simulink model "Drone_Formation"  (R2025a)
settings: Solver=FixedStepAuto  StartTime=0.0  StopTime=50  FixedStep=0.01  RelTol=1e-3
(part 1 of 2)
settings Model: Creator=huy01  LastModifiedBy=huy01

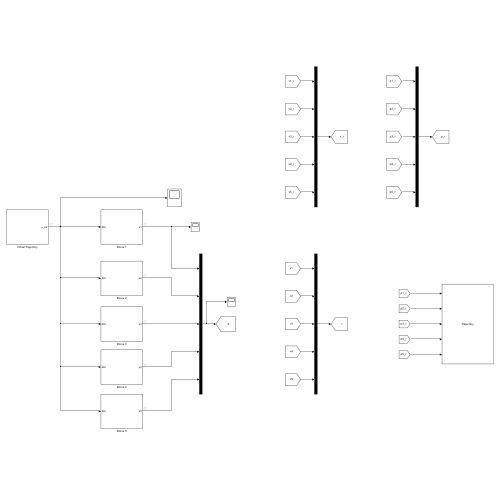
[thumbnail: Simulink's stored preview of the top-level diagram]
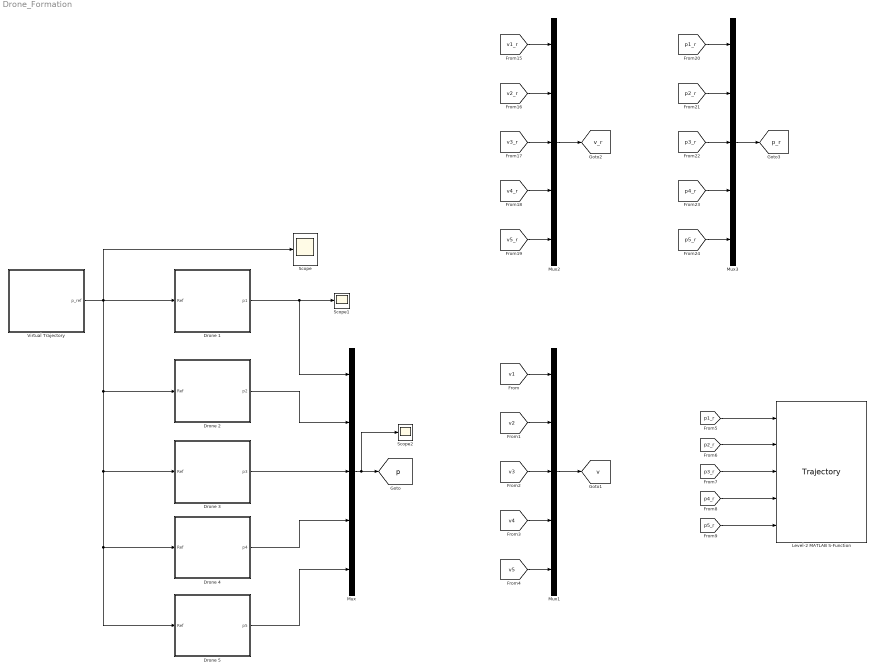
== system Drone_Formation ==
  Drone 1 : Subsystem
  Drone 2 : Subsystem
  Drone 3 : Subsystem
  Drone 4 : Subsystem
  Drone 5 : Subsystem
  Level-2 MATLAB S-Function : M-S-Function  FunctionName=Trajectory
  Mux{,1..3} (4 alike) : Mux  Inputs=5
  Scope : Scope
      settings: ActiveDisplayYMaximum=40
  Scope1 : Scope
      settings: ActiveDisplayYMinimum=-1380.4300146371204  ActiveDisplayYMaximum=836.3107963286418
  Scope2 : Scope
      settings: ActiveDisplayYMinimum=-1  ActiveDisplayYMaximum=1  DataLoggingVariableName=ScopeData2
  Virtual Trajectory : Subsystem
  tag scope: p=global, p_r=global, v=global, v_r=global
  wires:
  Virtual Trajectory/1(p_ref) -> Scope/1, Drone 1/1(Ref), Drone 2/1(Ref), Drone 5/1(Ref), Drone 4/1(Ref), Drone 3/1(Ref)
  Drone 3/1(p3) -> Mux/3
  Drone 4/1(p4) -> Mux/4
  Drone 5/1(p5) -> Mux/5
  Drone 1/1(p1) -> Scope1/1, Mux/1
  Drone 2/1(p2) -> Mux/2
  Mux/1 -> Scope2/1, [p]
  [v1] -> Mux1/1
  [v2] -> Mux1/2
  [v3] -> Mux1/3
  [v4] -> Mux1/4
  [v5] -> Mux1/5
  Mux1/1 -> [v]
  [p2_r] -> Level-2 MATLAB S-Function/2
  [p3_r] -> Level-2 MATLAB S-Function/3
  [p4_r] -> Level-2 MATLAB S-Function/4
  [p5_r] -> Level-2 MATLAB S-Function/5
  [p1_r] -> Level-2 MATLAB S-Function/1
  Mux2/1 -> [v_r]
  [v5_r] -> Mux2/5
  [v1_r] -> Mux2/1
  [v2_r] -> Mux2/2
  [v4_r] -> Mux2/4
  [v3_r] -> Mux2/3
  Mux3/1 -> [p_r]
  [p5_r] -> Mux3/5
  [p1_r] -> Mux3/1
  [p2_r] -> Mux3/2
  [p4_r] -> Mux3/4
  [p3_r] -> Mux3/3

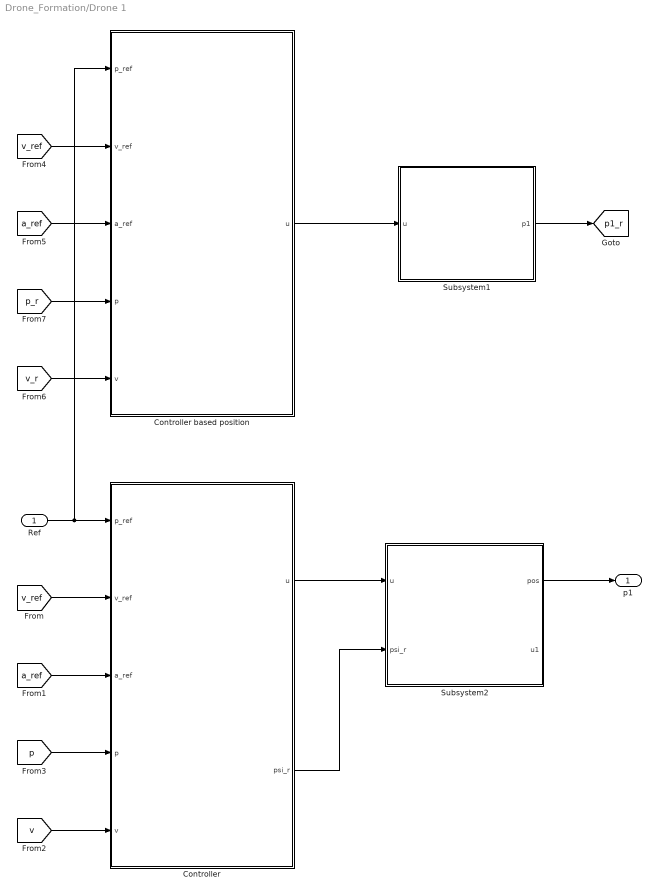
== system Drone_Formation/Drone 1 ==
  Ref : Inport
  Controller : MATLAB Function  TreatAsAtomicUnit=on
  Controller based position : MATLAB Function  TreatAsAtomicUnit=on
  Subsystem1 : Subsystem
  Subsystem2 : Subsystem
  p1 : Outport
  tag scope: p1_r=global
  wires:
  Ref/1 -> Controller based position/1(p_ref), Controller/1(p_ref)
  [v_ref] -> Controller/2(v_ref)
  [a_ref] -> Controller/3(a_ref)
  [v] -> Controller/5(v)
  [p] -> Controller/4(p)
  Controller/1(u) -> Subsystem2/1(u)
  Controller/2(psi_r) -> Subsystem2/2(psi_r)
  Subsystem2/1(pos) -> p1/1
  Subsystem1/1(p1) -> [p1_r]
  [a_ref] -> Controller based position/3(a_ref)
  [v_r] -> Controller based position/5(v)
  [p_r] -> Controller based position/4(p)
  Controller based position/1(u) -> Subsystem1/1(u)
  [v_ref] -> Controller based position/2(v_ref)

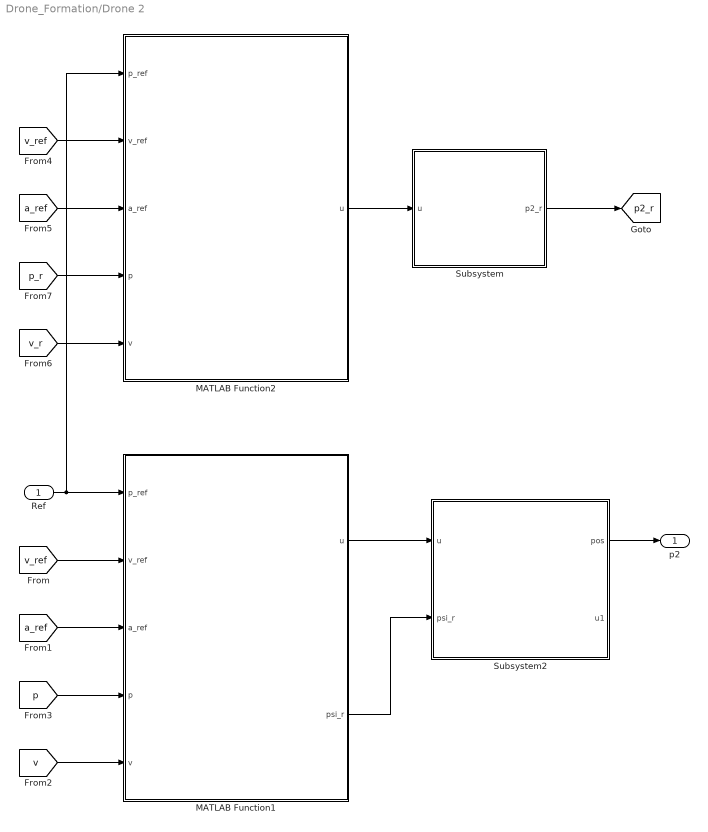
== system Drone_Formation/Drone 2 ==
  Ref : Inport
  MATLAB Function1 : MATLAB Function  TreatAsAtomicUnit=on
  MATLAB Function2 : MATLAB Function  TreatAsAtomicUnit=on
  Subsystem : Subsystem
  Subsystem2 : Subsystem
  p2 : Outport
  tag scope: p2_r=global
  wires:
  [v_ref] -> MATLAB Function1/2(v_ref)
  [a_ref] -> MATLAB Function1/3(a_ref)
  [v] -> MATLAB Function1/5(v)
  [p] -> MATLAB Function1/4(p)
  MATLAB Function1/1(u) -> Subsystem2/1(u)
  MATLAB Function1/2(psi_r) -> Subsystem2/2(psi_r)
  Subsystem2/1(pos) -> p2/1
  Subsystem/1(p2_r) -> [p2_r]
  MATLAB Function2/1(u) -> Subsystem/1(u)
  Ref/1 -> MATLAB Function2/1(p_ref), MATLAB Function1/1(p_ref)
  [v_ref] -> MATLAB Function2/2(v_ref)
  [v_r] -> MATLAB Function2/5(v)
  [p_r] -> MATLAB Function2/4(p)
  [a_ref] -> MATLAB Function2/3(a_ref)

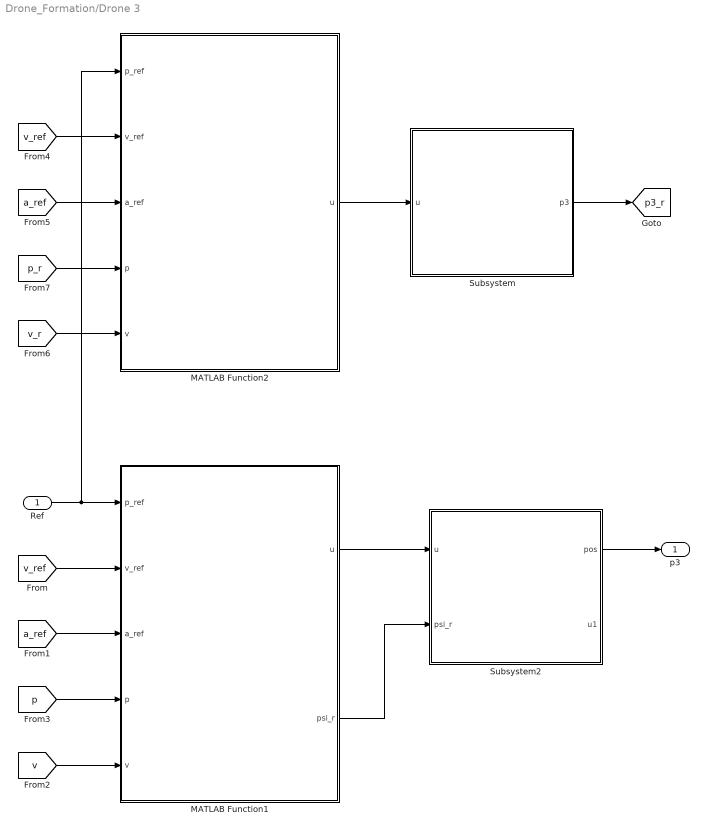
== system Drone_Formation/Drone 3 ==
  Ref : Inport
  MATLAB Function1 : MATLAB Function  TreatAsAtomicUnit=on
  MATLAB Function2 : MATLAB Function  TreatAsAtomicUnit=on
  Subsystem : Subsystem
  Subsystem2 : Subsystem
  p3 : Outport
  tag scope: p3_r=global
  wires:
  Ref/1 -> MATLAB Function2/1(p_ref), MATLAB Function1/1(p_ref)
  [v_ref] -> MATLAB Function1/2(v_ref)
  [a_ref] -> MATLAB Function1/3(a_ref)
  [v] -> MATLAB Function1/5(v)
  [p] -> MATLAB Function1/4(p)
  MATLAB Function1/1(u) -> Subsystem2/1(u)
  MATLAB Function1/2(psi_r) -> Subsystem2/2(psi_r)
  Subsystem2/1(pos) -> p3/1
  Subsystem/1(p3) -> [p3_r]
  [v_ref] -> MATLAB Function2/2(v_ref)
  [a_ref] -> MATLAB Function2/3(a_ref)
  [v_r] -> MATLAB Function2/5(v)
  [p_r] -> MATLAB Function2/4(p)
  MATLAB Function2/1(u) -> Subsystem/1(u)

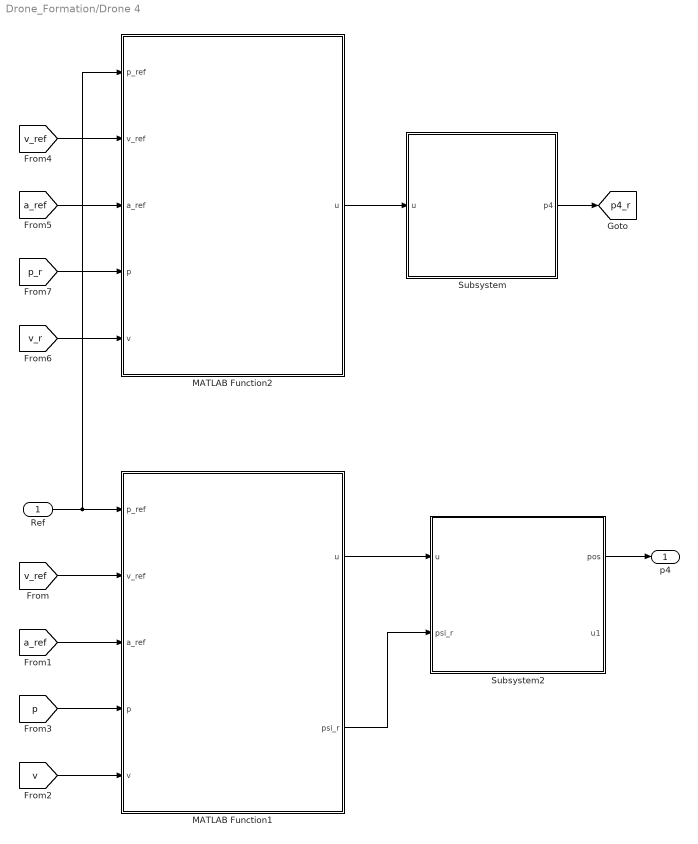
== system Drone_Formation/Drone 4 ==
  Ref : Inport
  MATLAB Function1 : MATLAB Function  TreatAsAtomicUnit=on
  MATLAB Function2 : MATLAB Function  TreatAsAtomicUnit=on
  Subsystem : Subsystem
  Subsystem2 : Subsystem
  p4 : Outport
  tag scope: p4_r=global
  wires:
  Ref/1 -> MATLAB Function2/1(p_ref), MATLAB Function1/1(p_ref)
  [v_ref] -> MATLAB Function1/2(v_ref)
  [a_ref] -> MATLAB Function1/3(a_ref)
  [v] -> MATLAB Function1/5(v)
  [p] -> MATLAB Function1/4(p)
  MATLAB Function1/1(u) -> Subsystem2/1(u)
  MATLAB Function1/2(psi_r) -> Subsystem2/2(psi_r)
  Subsystem2/1(pos) -> p4/1
  Subsystem/1(p4) -> [p4_r]
  [a_ref] -> MATLAB Function2/3(a_ref)
  [p_r] -> MATLAB Function2/4(p)
  [v_ref] -> MATLAB Function2/2(v_ref)
  [v_r] -> MATLAB Function2/5(v)
  MATLAB Function2/1(u) -> Subsystem/1(u)

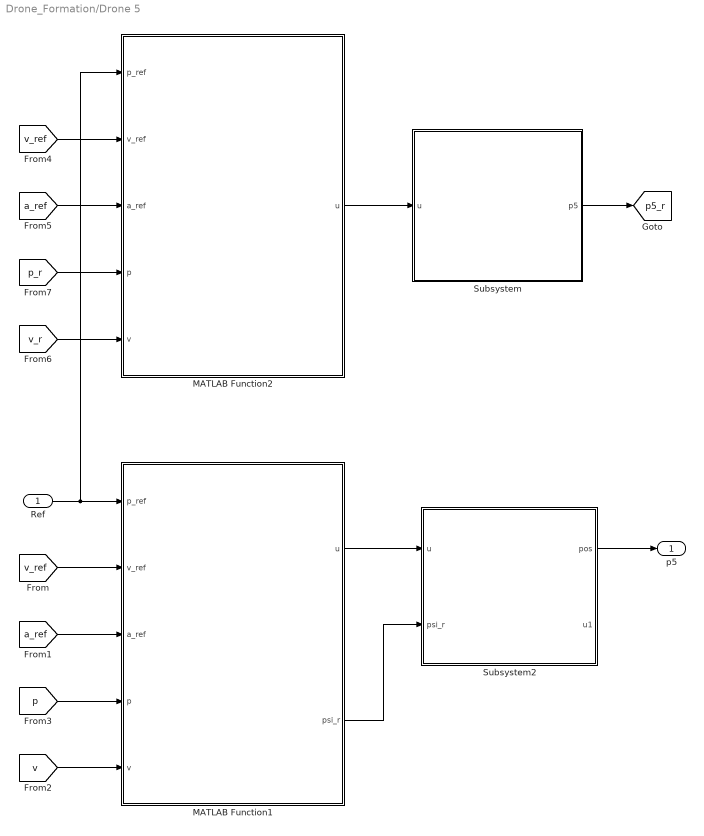
== system Drone_Formation/Drone 5 ==
  Ref : Inport
  MATLAB Function1 : MATLAB Function  TreatAsAtomicUnit=on
  MATLAB Function2 : MATLAB Function  TreatAsAtomicUnit=on
  Subsystem : Subsystem
  Subsystem2 : Subsystem
  p5 : Outport
  tag scope: p5_r=global
  wires:
  Ref/1 -> MATLAB Function2/1(p_ref), MATLAB Function1/1(p_ref)
  [v_ref] -> MATLAB Function1/2(v_ref)
  [a_ref] -> MATLAB Function1/3(a_ref)
  [v] -> MATLAB Function1/5(v)
  [p] -> MATLAB Function1/4(p)
  MATLAB Function1/1(u) -> Subsystem2/1(u)
  MATLAB Function1/2(psi_r) -> Subsystem2/2(psi_r)
  Subsystem2/1(pos) -> p5/1
  Subsystem/1(p5) -> [p5_r]
  [a_ref] -> MATLAB Function2/3(a_ref)
  [v_ref] -> MATLAB Function2/2(v_ref)
  [p_r] -> MATLAB Function2/4(p)
  [v_r] -> MATLAB Function2/5(v)
  MATLAB Function2/1(u) -> Subsystem/1(u)

== system Drone_Formation/Virtual Trajectory ==
  Clock : Clock
  Derivative : Derivative
  Derivative1 : Derivative
  MATLAB Function : MATLAB Function  TreatAsAtomicUnit=on
  p_ref : Outport
  tag scope: a_ref=global, v_ref=global
  wires:
  MATLAB Function/1(p_ref) -> Derivative/1, p_ref/1
  Clock/1 -> MATLAB Function/1(t)
  Derivative/1 -> Derivative1/1, [v_ref]
  Derivative1/1 -> [a_ref]

== system Drone_Formation/Drone 1/Subsystem1 ==
  u : Inport
  Integrator : Integrator  InitialCondition=zeros(3,1)
  Integrator1 : Integrator  InitialCondition=[4;5;0];
  Kinematic : MATLAB Function  TreatAsAtomicUnit=on
  p1 : Outport
  tag scope: v1_r=global
  wires:
  Integrator1/1 -> p1/1
  u/1 -> Kinematic/1(u)
  Integrator/1 -> [v1_r], Integrator1/1
  Kinematic/1(p1_ddot) -> Integrator/1

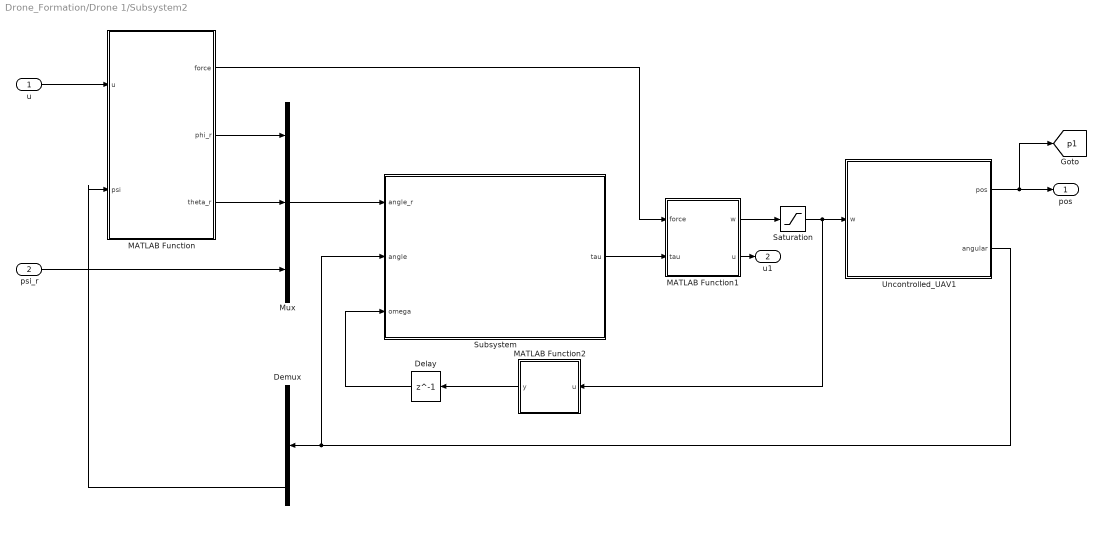
== system Drone_Formation/Drone 1/Subsystem2 ==
  u : Inport
  psi_r : Inport  Port=2
  Delay : Delay  DelayLength=1  InputProcessing=Columns as channels (frame based)
  Demux : Demux  Outputs=3
  MATLAB Function : MATLAB Function  TreatAsAtomicUnit=on
  MATLAB Function1 : MATLAB Function  TreatAsAtomicUnit=on
  MATLAB Function2 : MATLAB Function  TreatAsAtomicUnit=on
  Mux : Mux  Inputs=3
  Saturation : Saturate  UpperLimit=2300  LowerLimit=0
  Subsystem : Subsystem
  Uncontrolled_UAV1 : Subsystem
  pos : Outport
  u1 : Outport  Port=2
  tag scope: p1=global
  wires:
  MATLAB Function/2(phi_r) -> Mux/1
  Mux/1 -> Subsystem/1(angle_r)
  Uncontrolled_UAV1/2(angular) -> Subsystem/2(angle), Demux/1
  Saturation/1 -> Uncontrolled_UAV1/1(w), MATLAB Function2/1(u)
  MATLAB Function/3(theta_r) -> Mux/2
  Delay/1 -> Subsystem/3(omega)
  Subsystem/1(tau) -> MATLAB Function1/2(tau)
  psi_r/1 -> Mux/3
  MATLAB Function2/1(y) -> Delay/1
  MATLAB Function1/1(w) -> Saturation/1
  Demux/3 -> MATLAB Function/2(psi)
  MATLAB Function/1(force) -> MATLAB Function1/1(force)
  Uncontrolled_UAV1/1(pos) -> [p1], pos/1
  u/1 -> MATLAB Function/1(u)
  MATLAB Function1/2(u) -> u1/1

== system Drone_Formation/Drone 2/Subsystem ==
  u : Inport
  Integrator : Integrator  InitialCondition=zeros(3,1)
  Integrator1 : Integrator  InitialCondition=[5;1;0];
  Kinematic : MATLAB Function  TreatAsAtomicUnit=on
  p2_r : Outport
  tag scope: v2_r=global
  wires:
  Integrator/1 -> [v2_r], Integrator1/1
  Integrator1/1 -> p2_r/1
  u/1 -> Kinematic/1(u)
  Kinematic/1(p1_ddot) -> Integrator/1

== system Drone_Formation/Drone 2/Subsystem2 ==
  u : Inport
  psi_r : Inport  Port=2
  Delay : Delay  DelayLength=1  InputProcessing=Columns as channels (frame based)
  Demux : Demux  Outputs=3
  MATLAB Function : MATLAB Function  TreatAsAtomicUnit=on
  MATLAB Function1 : MATLAB Function  TreatAsAtomicUnit=on
  MATLAB Function2 : MATLAB Function  TreatAsAtomicUnit=on
  Mux : Mux  Inputs=3
  Saturation : Saturate  UpperLimit=2300  LowerLimit=0
  Subsystem : Subsystem
  Uncontrolled_UAV1 : Subsystem
  pos : Outport
  u1 : Outport  Port=2
  tag scope: p2=global
  wires:
  MATLAB Function/2(phi_r) -> Mux/1
  Mux/1 -> Subsystem/1(angle_r)
  Uncontrolled_UAV1/2(angular) -> Subsystem/2(angle), Demux/1
  Saturation/1 -> Uncontrolled_UAV1/1(w), MATLAB Function2/1(u)
  MATLAB Function/3(theta_r) -> Mux/2
  Delay/1 -> Subsystem/3(omega)
  Subsystem/1(tau) -> MATLAB Function1/2(tau)
  psi_r/1 -> Mux/3
  MATLAB Function2/1(y) -> Delay/1
  MATLAB Function1/1(w) -> Saturation/1
  Demux/3 -> MATLAB Function/2(psi)
  MATLAB Function/1(force) -> MATLAB Function1/1(force)
  Uncontrolled_UAV1/1(pos) -> [p2], pos/1
  u/1 -> MATLAB Function/1(u)
  MATLAB Function1/2(u) -> u1/1

== system Drone_Formation/Drone 3/Subsystem ==
  u : Inport
  Integrator : Integrator  InitialCondition=zeros(3,1)
  Integrator1 : Integrator  InitialCondition=zeros(3,1)
  Kinematic : MATLAB Function  TreatAsAtomicUnit=on
  p3 : Outport
  tag scope: v3_r=global
  wires:
  u/1 -> Kinematic/1(u)
  Integrator1/1 -> p3/1
  Integrator/1 -> [v3_r], Integrator1/1
  Kinematic/1(p1_ddot) -> Integrator/1

== system Drone_Formation/Drone 3/Subsystem2 ==
  u : Inport
  psi_r : Inport  Port=2
  Delay : Delay  DelayLength=1  InputProcessing=Columns as channels (frame based)
  Demux : Demux  Outputs=3
  MATLAB Function : MATLAB Function  TreatAsAtomicUnit=on
  MATLAB Function1 : MATLAB Function  TreatAsAtomicUnit=on
  MATLAB Function2 : MATLAB Function  TreatAsAtomicUnit=on
  Mux : Mux  Inputs=3
  Saturation : Saturate  UpperLimit=2300  LowerLimit=0
  Subsystem : Subsystem
  Uncontrolled_UAV1 : Subsystem
  pos : Outport
  u1 : Outport  Port=2
  tag scope: p3=global
  wires:
  MATLAB Function/2(phi_r) -> Mux/1
  Mux/1 -> Subsystem/1(angle_r)
  Uncontrolled_UAV1/2(angular) -> Subsystem/2(angle), Demux/1
  Saturation/1 -> Uncontrolled_UAV1/1(w), MATLAB Function2/1(u)
  MATLAB Function/3(theta_r) -> Mux/2
  Delay/1 -> Subsystem/3(omega)
  Subsystem/1(tau) -> MATLAB Function1/2(tau)
  psi_r/1 -> Mux/3
  MATLAB Function2/1(y) -> Delay/1
  MATLAB Function1/1(w) -> Saturation/1
  Demux/3 -> MATLAB Function/2(psi)
  MATLAB Function/1(force) -> MATLAB Function1/1(force)
  Uncontrolled_UAV1/1(pos) -> [p3], pos/1
  u/1 -> MATLAB Function/1(u)
  MATLAB Function1/2(u) -> u1/1

== system Drone_Formation/Drone 4/Subsystem ==
  u : Inport
  Integrator : Integrator  InitialCondition=zeros(3,1)
  Integrator1 : Integrator  InitialCondition=[10;2;0];
  Kinematic : MATLAB Function  TreatAsAtomicUnit=on
  p4 : Outport
  tag scope: v4_r=global
  wires:
  Integrator1/1 -> p4/1
  Integrator/1 -> [v4_r], Integrator1/1
  Kinematic/1(p1_ddot) -> Integrator/1
  u/1 -> Kinematic/1(u)

== system Drone_Formation/Drone 4/Subsystem2 ==
  u : Inport
  psi_r : Inport  Port=2
  Delay : Delay  DelayLength=1  InputProcessing=Columns as channels (frame based)
  Demux : Demux  Outputs=3
  MATLAB Function : MATLAB Function  TreatAsAtomicUnit=on
  MATLAB Function1 : MATLAB Function  TreatAsAtomicUnit=on
  MATLAB Function2 : MATLAB Function  TreatAsAtomicUnit=on
  Mux : Mux  Inputs=3
  Saturation : Saturate  UpperLimit=2300  LowerLimit=0
  Subsystem : Subsystem
  Uncontrolled_UAV1 : Subsystem
  pos : Outport
  u1 : Outport  Port=2
  tag scope: p4=global
  wires:
  MATLAB Function/2(phi_r) -> Mux/1
  Mux/1 -> Subsystem/1(angle_r)
  Uncontrolled_UAV1/2(angular) -> Subsystem/2(angle), Demux/1
  Saturation/1 -> Uncontrolled_UAV1/1(w), MATLAB Function2/1(u)
  MATLAB Function/3(theta_r) -> Mux/2
  Delay/1 -> Subsystem/3(omega)
  Subsystem/1(tau) -> MATLAB Function1/2(tau)
  psi_r/1 -> Mux/3
  MATLAB Function2/1(y) -> Delay/1
  MATLAB Function1/1(w) -> Saturation/1
  Demux/3 -> MATLAB Function/2(psi)
  MATLAB Function/1(force) -> MATLAB Function1/1(force)
  Uncontrolled_UAV1/1(pos) -> [p4], pos/1
  u/1 -> MATLAB Function/1(u)
  MATLAB Function1/2(u) -> u1/1

== system Drone_Formation/Drone 5/Subsystem ==
  u : Inport
  Integrator : Integrator  InitialCondition=zeros(3,1)
  Integrator1 : Integrator  InitialCondition=[15;0;0];
  Kinematic : MATLAB Function  TreatAsAtomicUnit=on
  p5 : Outport
  tag scope: v5_r=global
  wires:
  Integrator1/1 -> p5/1
  Kinematic/1(p1_ddot) -> Integrator/1
  Integrator/1 -> [v5_r], Integrator1/1
  u/1 -> Kinematic/1(u)

== system Drone_Formation/Drone 5/Subsystem2 ==
  u : Inport
  psi_r : Inport  Port=2
  Delay : Delay  DelayLength=1  InputProcessing=Columns as channels (frame based)
  Demux : Demux  Outputs=3
  MATLAB Function : MATLAB Function  TreatAsAtomicUnit=on
  MATLAB Function1 : MATLAB Function  TreatAsAtomicUnit=on
  MATLAB Function2 : MATLAB Function  TreatAsAtomicUnit=on
  Mux : Mux  Inputs=3
  Saturation : Saturate  UpperLimit=2300  LowerLimit=0
  Subsystem : Subsystem
  Uncontrolled_UAV1 : Subsystem
  pos : Outport
  u1 : Outport  Port=2
  tag scope: p5=global
  wires:
  MATLAB Function/2(phi_r) -> Mux/1
  Mux/1 -> Subsystem/1(angle_r)
  Uncontrolled_UAV1/2(angular) -> Subsystem/2(angle), Demux/1
  Saturation/1 -> Uncontrolled_UAV1/1(w), MATLAB Function2/1(u)
  MATLAB Function/3(theta_r) -> Mux/2
  Delay/1 -> Subsystem/3(omega)
  Subsystem/1(tau) -> MATLAB Function1/2(tau)
  psi_r/1 -> Mux/3
  MATLAB Function2/1(y) -> Delay/1
  MATLAB Function1/1(w) -> Saturation/1
  Demux/3 -> MATLAB Function/2(psi)
  MATLAB Function/1(force) -> MATLAB Function1/1(force)
  Uncontrolled_UAV1/1(pos) -> [p5], pos/1
  u/1 -> MATLAB Function/1(u)
  MATLAB Function1/2(u) -> u1/1

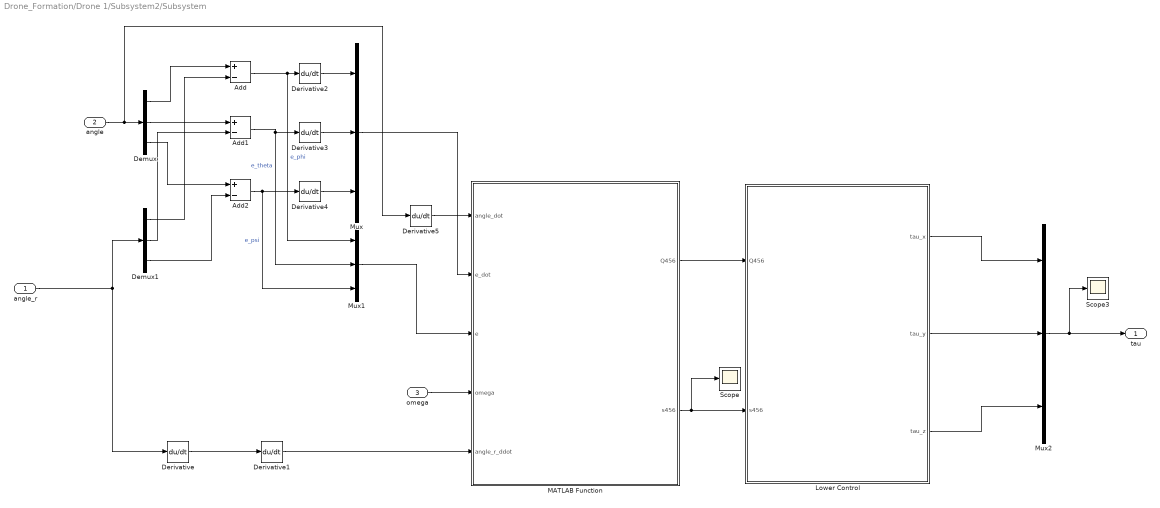
== system Drone_Formation/Drone 1/Subsystem2/Subsystem ==
  angle_r : Inport
  angle : Inport  Port=2
  omega : Inport  Port=3
  Add : Sum  Inputs=+-
  Add1 : Sum  Inputs=+-
  Add2 : Sum  Inputs=+-
  Demux : Demux  Outputs=3
  Demux1 : Demux  Outputs=3
  Derivative{,1..5} (6 alike) : Derivative
  Lower Control : MATLAB Function  TreatAsAtomicUnit=on
  MATLAB Function : MATLAB Function  TreatAsAtomicUnit=on
  Mux : Mux  Inputs=3
  Mux1 : Mux  Inputs=3
  Mux2 : Mux  Inputs=3
  Scope : Scope
      settings: ActiveDisplayYMinimum=-354.73382878164716  ActiveDisplayYMaximum=368.3791602340649  DataLoggingVariableName=ScopeData22
  Scope3 : Scope
      settings: ActiveDisplayYMinimum=-334.14921407033052  ActiveDisplayYMaximum=201.68653412472139  DataLoggingVariableName=ScopeData11
  tau : Outport
  wires:
  Add2/1 -> Mux1/3, Derivative4/1  "e_psi"
  Lower Control/2(tau_y) -> Mux2/2
  Mux1/1 -> MATLAB Function/3(e)
  Mux/1 -> MATLAB Function/2(e_dot)
  Mux2/1 -> tau/1, Scope3/1
  omega/1 -> MATLAB Function/4(omega)
  Add/1 -> Mux1/1, Derivative2/1  "e_phi"
  angle/1 -> Derivative5/1, Demux/1
  Derivative1/1 -> MATLAB Function/5(angle_r_ddot)
  MATLAB Function/1(Q456) -> Lower Control/1(Q456)
  Demux1/3 -> Add2/2
  Derivative3/1 -> Mux/2
  Demux/1 -> Add/1
  Lower Control/1(tau_x) -> Mux2/1
  Lower Control/3(tau_z) -> Mux2/3
  Demux1/1 -> Add/2
  angle_r/1 -> Demux1/1, Derivative/1
  Demux/2 -> Add1/1
  Add1/1 -> Mux1/2, Derivative3/1  "e_theta"
  Demux1/2 -> Add1/2
  Demux/3 -> Add2/1
  Derivative4/1 -> Mux/3
  Derivative/1 -> Derivative1/1
  Derivative2/1 -> Mux/1
  Derivative5/1 -> MATLAB Function/1(angle_dot)
  MATLAB Function/2(s456) -> Scope/1, Lower Control/2(s456)

== system Drone_Formation/Drone 1/Subsystem2/Uncontrolled_UAV1 ==
  w : Inport
  Delay : Delay  DelayLength=1  InputProcessing=Columns as channels (frame based)
  Demux : Demux
  MATLAB Function1 : MATLAB Function  TreatAsAtomicUnit=on
  Mux : Mux  Inputs=3
  Mux1 : Mux  Inputs=2
  Subsystem : Subsystem
  Subsystem1 : Subsystem
  pos : Outport
  angular : Outport  Port=2
  wires:
  w/1 -> Demux/1
  Demux/1 -> MATLAB Function1/1(w1)
  Demux/2 -> MATLAB Function1/2(w2)
  Demux/3 -> MATLAB Function1/3(w3)
  Demux/4 -> MATLAB Function1/4(w4)
  MATLAB Function1/3(tau_y) -> Mux/2
  MATLAB Function1/2(tau_x) -> Mux/1
  MATLAB Function1/4(tau_z) -> Mux/3
  Mux/1 -> Subsystem1/1(tau)
  Mux1/1 -> Subsystem/1(In1)
  Subsystem1/1(Out1) -> Mux1/2, angular/1
  MATLAB Function1/1(force) -> Mux1/1
  Subsystem/1(Out1) -> pos/1
  MATLAB Function1/5(omega) -> Delay/1
  Delay/1 -> Subsystem1/2(omega)

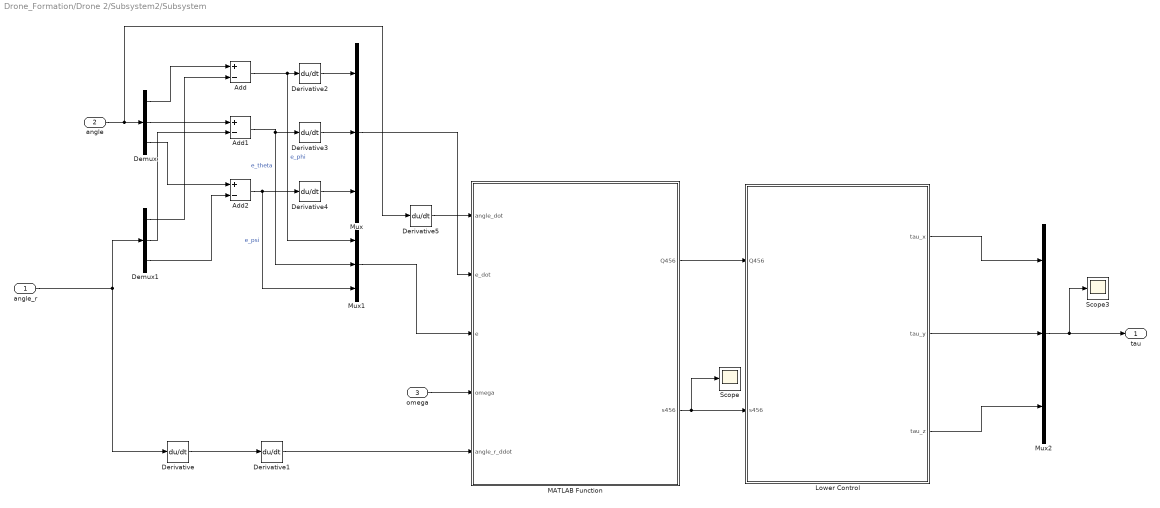
== system Drone_Formation/Drone 2/Subsystem2/Subsystem ==
  angle_r : Inport
  angle : Inport  Port=2
  omega : Inport  Port=3
  Add : Sum  Inputs=+-
  Add1 : Sum  Inputs=+-
  Add2 : Sum  Inputs=+-
  Demux : Demux  Outputs=3
  Demux1 : Demux  Outputs=3
  Derivative{,1..5} (6 alike) : Derivative
  Lower Control : MATLAB Function  TreatAsAtomicUnit=on
  MATLAB Function : MATLAB Function  TreatAsAtomicUnit=on
  Mux : Mux  Inputs=3
  Mux1 : Mux  Inputs=3
  Mux2 : Mux  Inputs=3
  Scope : Scope
      settings: ActiveDisplayYMinimum=-0.12582545562472158  ActiveDisplayYMaximum=0.10757646373161833  DataLoggingVariableName=ScopeData22
  Scope3 : Scope
      settings: ActiveDisplayYMinimum=-3.0869648432850987  ActiveDisplayYMaximum=4.3982035973405624  DataLoggingVariableName=ScopeData11
  tau : Outport
  wires:
  Add2/1 -> Mux1/3, Derivative4/1  "e_psi"
  Lower Control/2(tau_y) -> Mux2/2
  Mux1/1 -> MATLAB Function/3(e)
  Mux/1 -> MATLAB Function/2(e_dot)
  Mux2/1 -> tau/1, Scope3/1
  omega/1 -> MATLAB Function/4(omega)
  Add/1 -> Mux1/1, Derivative2/1  "e_phi"
  angle/1 -> Derivative5/1, Demux/1
  Derivative1/1 -> MATLAB Function/5(angle_r_ddot)
  MATLAB Function/1(Q456) -> Lower Control/1(Q456)
  Demux1/3 -> Add2/2
  Derivative3/1 -> Mux/2
  Demux/1 -> Add/1
  Lower Control/1(tau_x) -> Mux2/1
  Lower Control/3(tau_z) -> Mux2/3
  Demux1/1 -> Add/2
  angle_r/1 -> Demux1/1, Derivative/1
  Demux/2 -> Add1/1
  Add1/1 -> Mux1/2, Derivative3/1  "e_theta"
  Demux1/2 -> Add1/2
  Demux/3 -> Add2/1
  Derivative4/1 -> Mux/3
  Derivative/1 -> Derivative1/1
  Derivative2/1 -> Mux/1
  Derivative5/1 -> MATLAB Function/1(angle_dot)
  MATLAB Function/2(s456) -> Scope/1, Lower Control/2(s456)

== system Drone_Formation/Drone 2/Subsystem2/Uncontrolled_UAV1 ==
  w : Inport
  Delay : Delay  DelayLength=1  InputProcessing=Columns as channels (frame based)
  Demux : Demux
  MATLAB Function1 : MATLAB Function  TreatAsAtomicUnit=on
  Mux : Mux  Inputs=3
  Mux1 : Mux  Inputs=2
  Subsystem : Subsystem
  Subsystem1 : Subsystem
  pos : Outport
  angular : Outport  Port=2
  wires:
  w/1 -> Demux/1
  Demux/1 -> MATLAB Function1/1(w1)
  Demux/2 -> MATLAB Function1/2(w2)
  Demux/3 -> MATLAB Function1/3(w3)
  Demux/4 -> MATLAB Function1/4(w4)
  MATLAB Function1/3(tau_y) -> Mux/2
  MATLAB Function1/2(tau_x) -> Mux/1
  MATLAB Function1/4(tau_z) -> Mux/3
  Mux/1 -> Subsystem1/1(tau)
  Mux1/1 -> Subsystem/1(In1)
  Subsystem1/1(Out1) -> Mux1/2, angular/1
  MATLAB Function1/1(force) -> Mux1/1
  Subsystem/1(Out1) -> pos/1
  MATLAB Function1/5(omega) -> Delay/1
  Delay/1 -> Subsystem1/2(omega)

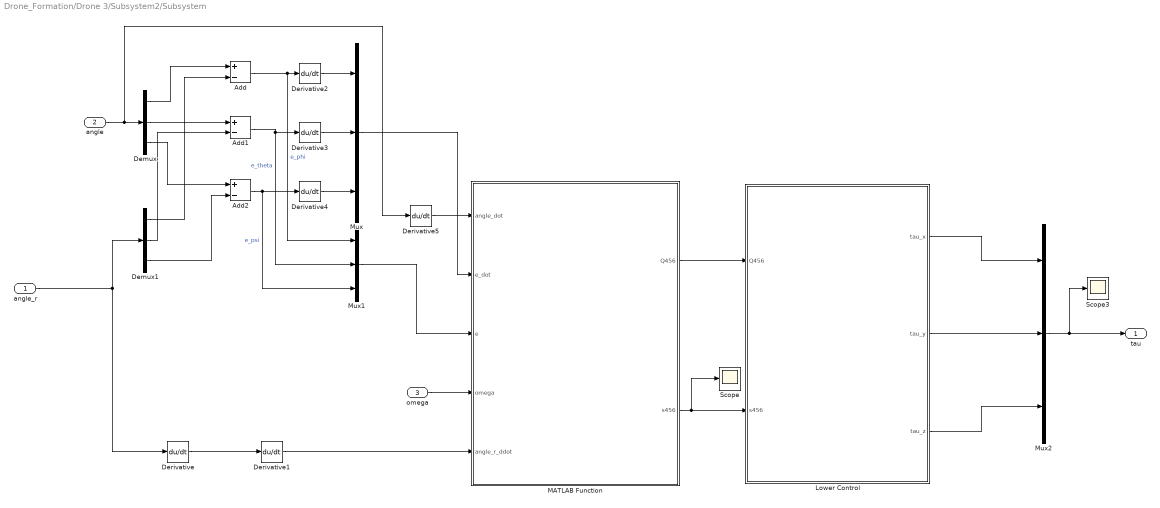
== system Drone_Formation/Drone 3/Subsystem2/Subsystem ==
  angle_r : Inport
  angle : Inport  Port=2
  omega : Inport  Port=3
  Add : Sum  Inputs=+-
  Add1 : Sum  Inputs=+-
  Add2 : Sum  Inputs=+-
  Demux : Demux  Outputs=3
  Demux1 : Demux  Outputs=3
  Derivative{,1..5} (6 alike) : Derivative
  Lower Control : MATLAB Function  TreatAsAtomicUnit=on
  MATLAB Function : MATLAB Function  TreatAsAtomicUnit=on
  Mux : Mux  Inputs=3
  Mux1 : Mux  Inputs=3
  Mux2 : Mux  Inputs=3
  Scope : Scope
      settings: ActiveDisplayYMinimum=-0.12582545562472158  ActiveDisplayYMaximum=0.10757646373161833  DataLoggingVariableName=ScopeData22
  Scope3 : Scope
      settings: ActiveDisplayYMinimum=-3.0869648432850987  ActiveDisplayYMaximum=4.3982035973405624  DataLoggingVariableName=ScopeData11
  tau : Outport
  wires:
  Add2/1 -> Mux1/3, Derivative4/1  "e_psi"
  Lower Control/2(tau_y) -> Mux2/2
  Mux1/1 -> MATLAB Function/3(e)
  Mux/1 -> MATLAB Function/2(e_dot)
  Mux2/1 -> tau/1, Scope3/1
  omega/1 -> MATLAB Function/4(omega)
  Add/1 -> Mux1/1, Derivative2/1  "e_phi"
  angle/1 -> Derivative5/1, Demux/1
  Derivative1/1 -> MATLAB Function/5(angle_r_ddot)
  MATLAB Function/1(Q456) -> Lower Control/1(Q456)
  Demux1/3 -> Add2/2
  Derivative3/1 -> Mux/2
  Demux/1 -> Add/1
  Lower Control/1(tau_x) -> Mux2/1
  Lower Control/3(tau_z) -> Mux2/3
  Demux1/1 -> Add/2
  angle_r/1 -> Demux1/1, Derivative/1
  Demux/2 -> Add1/1
  Add1/1 -> Mux1/2, Derivative3/1  "e_theta"
  Demux1/2 -> Add1/2
  Demux/3 -> Add2/1
  Derivative4/1 -> Mux/3
  Derivative/1 -> Derivative1/1
  Derivative2/1 -> Mux/1
  Derivative5/1 -> MATLAB Function/1(angle_dot)
  MATLAB Function/2(s456) -> Scope/1, Lower Control/2(s456)

== system Drone_Formation/Drone 3/Subsystem2/Uncontrolled_UAV1 ==
  w : Inport
  Delay : Delay  DelayLength=1  InputProcessing=Columns as channels (frame based)
  Demux : Demux
  MATLAB Function1 : MATLAB Function  TreatAsAtomicUnit=on
  Mux : Mux  Inputs=3
  Mux1 : Mux  Inputs=2
  Subsystem : Subsystem
  Subsystem1 : Subsystem
  pos : Outport
  angular : Outport  Port=2
  wires:
  w/1 -> Demux/1
  Demux/1 -> MATLAB Function1/1(w1)
  Demux/2 -> MATLAB Function1/2(w2)
  Demux/3 -> MATLAB Function1/3(w3)
  Demux/4 -> MATLAB Function1/4(w4)
  MATLAB Function1/3(tau_y) -> Mux/2
  MATLAB Function1/2(tau_x) -> Mux/1
  MATLAB Function1/4(tau_z) -> Mux/3
  Mux/1 -> Subsystem1/1(tau)
  Mux1/1 -> Subsystem/1(In1)
  Subsystem1/1(Out1) -> Mux1/2, angular/1
  MATLAB Function1/1(force) -> Mux1/1
  Subsystem/1(Out1) -> pos/1
  MATLAB Function1/5(omega) -> Delay/1
  Delay/1 -> Subsystem1/2(omega)

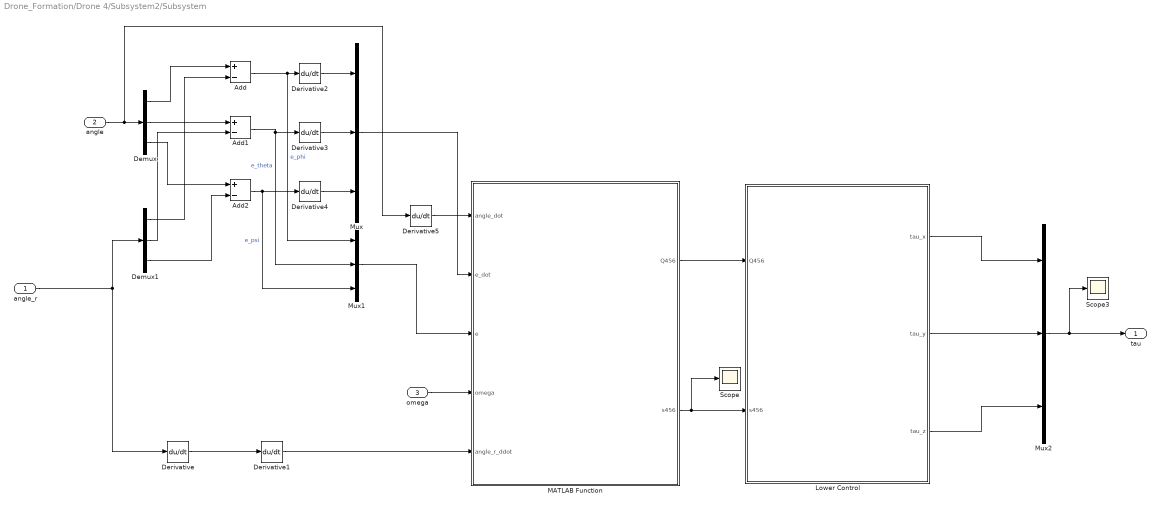
== system Drone_Formation/Drone 4/Subsystem2/Subsystem ==
  angle_r : Inport
  angle : Inport  Port=2
  omega : Inport  Port=3
  Add : Sum  Inputs=+-
  Add1 : Sum  Inputs=+-
  Add2 : Sum  Inputs=+-
  Demux : Demux  Outputs=3
  Demux1 : Demux  Outputs=3
  Derivative{,1..5} (6 alike) : Derivative
  Lower Control : MATLAB Function  TreatAsAtomicUnit=on
  MATLAB Function : MATLAB Function  TreatAsAtomicUnit=on
  Mux : Mux  Inputs=3
  Mux1 : Mux  Inputs=3
  Mux2 : Mux  Inputs=3
  Scope : Scope
      settings: ActiveDisplayYMinimum=-0.12582545562472158  ActiveDisplayYMaximum=0.10757646373161833  DataLoggingVariableName=ScopeData22
  Scope3 : Scope
      settings: ActiveDisplayYMinimum=-3.0869648432850987  ActiveDisplayYMaximum=4.3982035973405624  DataLoggingVariableName=ScopeData11
  tau : Outport
  wires:
  Add2/1 -> Mux1/3, Derivative4/1  "e_psi"
  Lower Control/2(tau_y) -> Mux2/2
  Mux1/1 -> MATLAB Function/3(e)
  Mux/1 -> MATLAB Function/2(e_dot)
  Mux2/1 -> tau/1, Scope3/1
  omega/1 -> MATLAB Function/4(omega)
  Add/1 -> Mux1/1, Derivative2/1  "e_phi"
  angle/1 -> Derivative5/1, Demux/1
  Derivative1/1 -> MATLAB Function/5(angle_r_ddot)
  MATLAB Function/1(Q456) -> Lower Control/1(Q456)
  Demux1/3 -> Add2/2
  Derivative3/1 -> Mux/2
  Demux/1 -> Add/1
  Lower Control/1(tau_x) -> Mux2/1
  Lower Control/3(tau_z) -> Mux2/3
  Demux1/1 -> Add/2
  angle_r/1 -> Demux1/1, Derivative/1
  Demux/2 -> Add1/1
  Add1/1 -> Mux1/2, Derivative3/1  "e_theta"
  Demux1/2 -> Add1/2
  Demux/3 -> Add2/1
  Derivative4/1 -> Mux/3
  Derivative/1 -> Derivative1/1
  Derivative2/1 -> Mux/1
  Derivative5/1 -> MATLAB Function/1(angle_dot)
  MATLAB Function/2(s456) -> Scope/1, Lower Control/2(s456)

== system Drone_Formation/Drone 4/Subsystem2/Uncontrolled_UAV1 ==
  w : Inport
  Delay : Delay  DelayLength=1  InputProcessing=Columns as channels (frame based)
  Demux : Demux
  MATLAB Function1 : MATLAB Function  TreatAsAtomicUnit=on
  Mux : Mux  Inputs=3
  Mux1 : Mux  Inputs=2
  Subsystem : Subsystem
  Subsystem1 : Subsystem
  pos : Outport
  angular : Outport  Port=2
  wires:
  w/1 -> Demux/1
  Demux/1 -> MATLAB Function1/1(w1)
  Demux/2 -> MATLAB Function1/2(w2)
  Demux/3 -> MATLAB Function1/3(w3)
  Demux/4 -> MATLAB Function1/4(w4)
  MATLAB Function1/3(tau_y) -> Mux/2
  MATLAB Function1/2(tau_x) -> Mux/1
  MATLAB Function1/4(tau_z) -> Mux/3
  Mux/1 -> Subsystem1/1(tau)
  Mux1/1 -> Subsystem/1(In1)
  Subsystem1/1(Out1) -> Mux1/2, angular/1
  MATLAB Function1/1(force) -> Mux1/1
  Subsystem/1(Out1) -> pos/1
  MATLAB Function1/5(omega) -> Delay/1
  Delay/1 -> Subsystem1/2(omega)

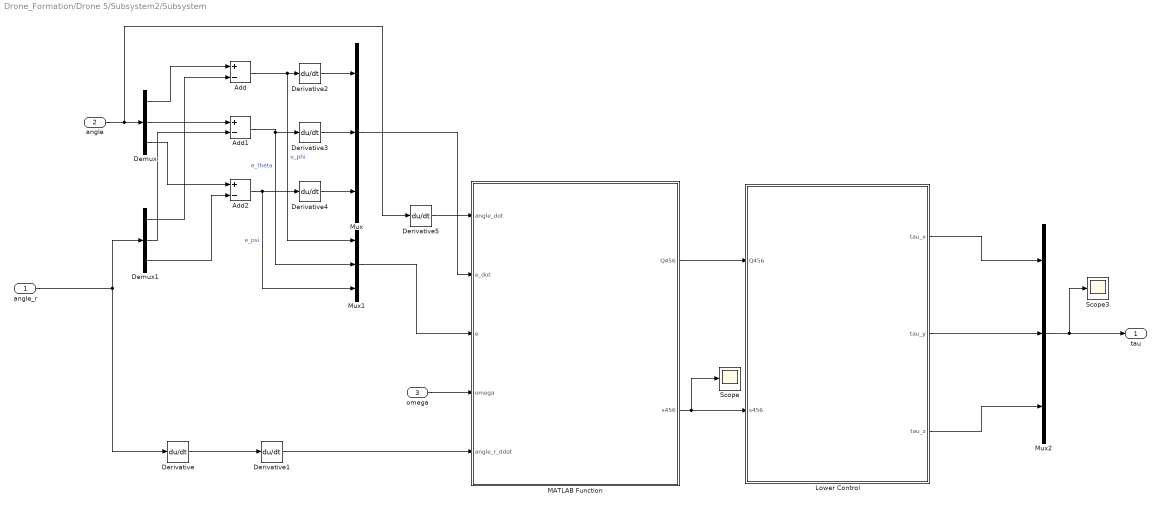
== system Drone_Formation/Drone 5/Subsystem2/Subsystem ==
  angle_r : Inport
  angle : Inport  Port=2
  omega : Inport  Port=3
  Add : Sum  Inputs=+-
  Add1 : Sum  Inputs=+-
  Add2 : Sum  Inputs=+-
  Demux : Demux  Outputs=3
  Demux1 : Demux  Outputs=3
  Derivative{,1..5} (6 alike) : Derivative
  Lower Control : MATLAB Function  TreatAsAtomicUnit=on
  MATLAB Function : MATLAB Function  TreatAsAtomicUnit=on
  Mux : Mux  Inputs=3
  Mux1 : Mux  Inputs=3
  Mux2 : Mux  Inputs=3
  Scope : Scope
      settings: ActiveDisplayYMinimum=-0.12582545562472158  ActiveDisplayYMaximum=0.10757646373161833  DataLoggingVariableName=ScopeData22
  Scope3 : Scope
      settings: ActiveDisplayYMinimum=-3.0869648432850987  ActiveDisplayYMaximum=4.3982035973405624  DataLoggingVariableName=ScopeData11
  tau : Outport
  wires:
  Add2/1 -> Mux1/3, Derivative4/1  "e_psi"
  Lower Control/2(tau_y) -> Mux2/2
  Mux1/1 -> MATLAB Function/3(e)
  Mux/1 -> MATLAB Function/2(e_dot)
  Mux2/1 -> tau/1, Scope3/1
  omega/1 -> MATLAB Function/4(omega)
  Add/1 -> Mux1/1, Derivative2/1  "e_phi"
  angle/1 -> Derivative5/1, Demux/1
  Derivative1/1 -> MATLAB Function/5(angle_r_ddot)
  MATLAB Function/1(Q456) -> Lower Control/1(Q456)
  Demux1/3 -> Add2/2
  Derivative3/1 -> Mux/2
  Demux/1 -> Add/1
  Lower Control/1(tau_x) -> Mux2/1
  Lower Control/3(tau_z) -> Mux2/3
  Demux1/1 -> Add/2
  angle_r/1 -> Demux1/1, Derivative/1
  Demux/2 -> Add1/1
  Add1/1 -> Mux1/2, Derivative3/1  "e_theta"
  Demux1/2 -> Add1/2
  Demux/3 -> Add2/1
  Derivative4/1 -> Mux/3
  Derivative/1 -> Derivative1/1
  Derivative2/1 -> Mux/1
  Derivative5/1 -> MATLAB Function/1(angle_dot)
  MATLAB Function/2(s456) -> Scope/1, Lower Control/2(s456)

== system Drone_Formation/Drone 5/Subsystem2/Uncontrolled_UAV1 ==
  w : Inport
  Delay : Delay  DelayLength=1  InputProcessing=Columns as channels (frame based)
  Demux : Demux
  MATLAB Function1 : MATLAB Function  TreatAsAtomicUnit=on
  Mux : Mux  Inputs=3
  Mux1 : Mux  Inputs=2
  Subsystem : Subsystem
  Subsystem1 : Subsystem
  pos : Outport
  angular : Outport  Port=2
  wires:
  w/1 -> Demux/1
  Demux/1 -> MATLAB Function1/1(w1)
  Demux/2 -> MATLAB Function1/2(w2)
  Demux/3 -> MATLAB Function1/3(w3)
  Demux/4 -> MATLAB Function1/4(w4)
  MATLAB Function1/3(tau_y) -> Mux/2
  MATLAB Function1/2(tau_x) -> Mux/1
  MATLAB Function1/4(tau_z) -> Mux/3
  Mux/1 -> Subsystem1/1(tau)
  Mux1/1 -> Subsystem/1(In1)
  Subsystem1/1(Out1) -> Mux1/2, angular/1
  MATLAB Function1/1(force) -> Mux1/1
  Subsystem/1(Out1) -> pos/1
  MATLAB Function1/5(omega) -> Delay/1
  Delay/1 -> Subsystem1/2(omega)

== system Drone_Formation/Drone 1/Subsystem2/Uncontrolled_UAV1/Subsystem ==
  In1 : Inport
  Demux1 : Demux
  Integrator{,1..2,4} (4 alike) : Integrator
  Integrator3 : Integrator  InitialCondition=-2
  Integrator5 : Integrator  InitialCondition=1
  MATLAB Function : MATLAB Function  TreatAsAtomicUnit=on
  Mux : Mux  Inputs=3
  Mux1 : Mux  Inputs=3
  Scope1 : Scope
      settings: ActiveDisplayYMinimum=-53.661197596804719  ActiveDisplayYMaximum=492.95077837124262  DataLoggingVariableName=ScopeData3
  Out1 : Outport
  tag scope: v1=global
  wires:
  Demux1/3 -> MATLAB Function/3(theta)
  Integrator/1 -> Mux1/1, Integrator3/1
  Demux1/4 -> MATLAB Function/4(psi)
  Demux1/1 -> MATLAB Function/1(force)
  Demux1/2 -> MATLAB Function/2(phi)
  In1/1 -> Demux1/1
  MATLAB Function/1(x_ddot) -> Integrator/1
  MATLAB Function/2(y_ddot) -> Integrator1/1
  Integrator1/1 -> Mux1/2, Integrator4/1
  MATLAB Function/3(z_ddot) -> Integrator2/1
  Integrator2/1 -> Mux1/3, Integrator5/1
  Mux/1 -> Out1/1
  Integrator4/1 -> Mux/2
  Integrator3/1 -> Mux/1
  Integrator5/1 -> Mux/3, Scope1/1
  Mux1/1 -> [v1]

== system Drone_Formation/Drone 1/Subsystem2/Uncontrolled_UAV1/Subsystem1 ==
  tau : Inport
  omega : Inport  Port=2
  Integrator{,1..2,5} (4 alike) : Integrator
  Integrator3 : Integrator  InitialCondition=pi/4
  Integrator4 : Integrator  InitialCondition=pi/6
  MATLAB Function : MATLAB Function  TreatAsAtomicUnit=on
  Mux : Mux  Inputs=3
  Out1 : Outport
  wires:
  MATLAB Function/1(phi_ddot) -> Integrator/1
  tau/1 -> MATLAB Function/1(tau)
  MATLAB Function/2(theta_ddot) -> Integrator1/1
  MATLAB Function/3(psi_ddot) -> Integrator2/1
  Integrator/1 -> Integrator3/1, MATLAB Function/2(phi_dot)
  Integrator1/1 -> Integrator4/1, MATLAB Function/3(theta_dot)
  Integrator2/1 -> Integrator5/1, MATLAB Function/4(psi_dot)
  Integrator4/1 -> Mux/2  "theta"
  Integrator3/1 -> Mux/1  "phi"
  Integrator5/1 -> Mux/3  "psi"
  Mux/1 -> Out1/1
  omega/1 -> MATLAB Function/5(omega)

== system Drone_Formation/Drone 2/Subsystem2/Uncontrolled_UAV1/Subsystem ==
  In1 : Inport
  Demux1 : Demux
  Integrator{,1..2,4} (4 alike) : Integrator
  Integrator3 : Integrator  InitialCondition=-2
  Integrator5 : Integrator  InitialCondition=1
  MATLAB Function : MATLAB Function  TreatAsAtomicUnit=on
  Mux : Mux  Inputs=3
  Mux1 : Mux  Inputs=3
  Scope1 : Scope
      settings: ActiveDisplayYMinimum=-53.661197596804719  ActiveDisplayYMaximum=492.95077837124262  DataLoggingVariableName=ScopeData3
  Out1 : Outport
  tag scope: v2=global
  wires:
  Demux1/3 -> MATLAB Function/3(theta)
  Integrator/1 -> Mux1/1, Integrator3/1
  Demux1/4 -> MATLAB Function/4(psi)
  Demux1/1 -> MATLAB Function/1(force)
  Demux1/2 -> MATLAB Function/2(phi)
  In1/1 -> Demux1/1
  MATLAB Function/1(x_ddot) -> Integrator/1
  MATLAB Function/2(y_ddot) -> Integrator1/1
  Integrator1/1 -> Mux1/2, Integrator4/1
  MATLAB Function/3(z_ddot) -> Integrator2/1
  Integrator2/1 -> Mux1/3, Integrator5/1
  Mux/1 -> Out1/1
  Integrator4/1 -> Mux/2
  Integrator3/1 -> Mux/1
  Integrator5/1 -> Mux/3, Scope1/1
  Mux1/1 -> [v2]

== system Drone_Formation/Drone 2/Subsystem2/Uncontrolled_UAV1/Subsystem1 ==
  tau : Inport
  omega : Inport  Port=2
  Integrator{,1..2,5} (4 alike) : Integrator
  Integrator3 : Integrator  InitialCondition=pi/4
  Integrator4 : Integrator  InitialCondition=pi/6
  MATLAB Function : MATLAB Function  TreatAsAtomicUnit=on
  Mux : Mux  Inputs=3
  Out1 : Outport
  wires:
  MATLAB Function/1(phi_ddot) -> Integrator/1
  tau/1 -> MATLAB Function/1(tau)
  MATLAB Function/2(theta_ddot) -> Integrator1/1
  MATLAB Function/3(psi_ddot) -> Integrator2/1
  Integrator/1 -> Integrator3/1, MATLAB Function/2(phi_dot)
  Integrator1/1 -> Integrator4/1, MATLAB Function/3(theta_dot)
  Integrator2/1 -> Integrator5/1, MATLAB Function/4(psi_dot)
  Integrator4/1 -> Mux/2  "theta"
  Integrator3/1 -> Mux/1  "phi"
  Integrator5/1 -> Mux/3  "psi"
  Mux/1 -> Out1/1
  omega/1 -> MATLAB Function/5(omega)

== system Drone_Formation/Drone 3/Subsystem2/Uncontrolled_UAV1/Subsystem ==
  In1 : Inport
  Demux1 : Demux
  Integrator{,1..2,4} (4 alike) : Integrator
  Integrator3 : Integrator  InitialCondition=-2
  Integrator5 : Integrator  InitialCondition=1
  MATLAB Function : MATLAB Function  TreatAsAtomicUnit=on
  Mux : Mux  Inputs=3
  Mux1 : Mux  Inputs=3
  Scope1 : Scope
      settings: ActiveDisplayYMinimum=-53.661197596804719  ActiveDisplayYMaximum=492.95077837124262  DataLoggingVariableName=ScopeData3
  Out1 : Outport
  tag scope: v3=global
  wires:
  Demux1/3 -> MATLAB Function/3(theta)
  Integrator/1 -> Mux1/1, Integrator3/1
  Demux1/4 -> MATLAB Function/4(psi)
  Demux1/1 -> MATLAB Function/1(force)
  Demux1/2 -> MATLAB Function/2(phi)
  In1/1 -> Demux1/1
  MATLAB Function/1(x_ddot) -> Integrator/1
  MATLAB Function/2(y_ddot) -> Integrator1/1
  Integrator1/1 -> Mux1/2, Integrator4/1
  MATLAB Function/3(z_ddot) -> Integrator2/1
  Integrator2/1 -> Mux1/3, Integrator5/1
  Mux/1 -> Out1/1
  Integrator4/1 -> Mux/2
  Integrator3/1 -> Mux/1
  Integrator5/1 -> Mux/3, Scope1/1
  Mux1/1 -> [v3]

== system Drone_Formation/Drone 3/Subsystem2/Uncontrolled_UAV1/Subsystem1 ==
  tau : Inport
  omega : Inport  Port=2
  Integrator{,1..2,5} (4 alike) : Integrator
  Integrator3 : Integrator  InitialCondition=pi/4
  Integrator4 : Integrator  InitialCondition=pi/6
  MATLAB Function : MATLAB Function  TreatAsAtomicUnit=on
  Mux : Mux  Inputs=3
  Out1 : Outport
  wires:
  MATLAB Function/1(phi_ddot) -> Integrator/1
  tau/1 -> MATLAB Function/1(tau)
  MATLAB Function/2(theta_ddot) -> Integrator1/1
  MATLAB Function/3(psi_ddot) -> Integrator2/1
  Integrator/1 -> Integrator3/1, MATLAB Function/2(phi_dot)
  Integrator1/1 -> Integrator4/1, MATLAB Function/3(theta_dot)
  Integrator2/1 -> Integrator5/1, MATLAB Function/4(psi_dot)
  Integrator4/1 -> Mux/2  "theta"
  Integrator3/1 -> Mux/1  "phi"
  Integrator5/1 -> Mux/3  "psi"
  Mux/1 -> Out1/1
  omega/1 -> MATLAB Function/5(omega)

== system Drone_Formation/Drone 4/Subsystem2/Uncontrolled_UAV1/Subsystem ==
  In1 : Inport
  Demux1 : Demux
  Integrator{,1..2,4} (4 alike) : Integrator
  Integrator3 : Integrator  InitialCondition=-2
  Integrator5 : Integrator  InitialCondition=1
  MATLAB Function : MATLAB Function  TreatAsAtomicUnit=on
  Mux : Mux  Inputs=3
  Mux1 : Mux  Inputs=3
  Scope1 : Scope
      settings: ActiveDisplayYMinimum=-53.661197596804719  ActiveDisplayYMaximum=492.95077837124262  DataLoggingVariableName=ScopeData3
  Out1 : Outport
  tag scope: v4=global
  wires:
  Demux1/3 -> MATLAB Function/3(theta)
  Integrator/1 -> Mux1/1, Integrator3/1
  Demux1/4 -> MATLAB Function/4(psi)
  Demux1/1 -> MATLAB Function/1(force)
  Demux1/2 -> MATLAB Function/2(phi)
  In1/1 -> Demux1/1
  MATLAB Function/1(x_ddot) -> Integrator/1
  MATLAB Function/2(y_ddot) -> Integrator1/1
  Integrator1/1 -> Mux1/2, Integrator4/1
  MATLAB Function/3(z_ddot) -> Integrator2/1
  Integrator2/1 -> Mux1/3, Integrator5/1
  Mux/1 -> Out1/1
  Integrator4/1 -> Mux/2
  Integrator3/1 -> Mux/1
  Integrator5/1 -> Mux/3, Scope1/1
  Mux1/1 -> [v4]

== system Drone_Formation/Drone 4/Subsystem2/Uncontrolled_UAV1/Subsystem1 ==
  tau : Inport
  omega : Inport  Port=2
  Integrator{,1..2,5} (4 alike) : Integrator
  Integrator3 : Integrator  InitialCondition=pi/4
  Integrator4 : Integrator  InitialCondition=pi/6
  MATLAB Function : MATLAB Function  TreatAsAtomicUnit=on
  Mux : Mux  Inputs=3
  Out1 : Outport
  wires:
  MATLAB Function/1(phi_ddot) -> Integrator/1
  tau/1 -> MATLAB Function/1(tau)
  MATLAB Function/2(theta_ddot) -> Integrator1/1
  MATLAB Function/3(psi_ddot) -> Integrator2/1
  Integrator/1 -> Integrator3/1, MATLAB Function/2(phi_dot)
  Integrator1/1 -> Integrator4/1, MATLAB Function/3(theta_dot)
  Integrator2/1 -> Integrator5/1, MATLAB Function/4(psi_dot)
  Integrator4/1 -> Mux/2  "theta"
  Integrator3/1 -> Mux/1  "phi"
  Integrator5/1 -> Mux/3  "psi"
  Mux/1 -> Out1/1
  omega/1 -> MATLAB Function/5(omega)

== system Drone_Formation/Drone 5/Subsystem2/Uncontrolled_UAV1/Subsystem ==
  In1 : Inport
  Demux1 : Demux
  Integrator{,1..2,4} (4 alike) : Integrator
  Integrator3 : Integrator  InitialCondition=-2
  Integrator5 : Integrator  InitialCondition=1
  MATLAB Function : MATLAB Function  TreatAsAtomicUnit=on
  Mux : Mux  Inputs=3
  Mux1 : Mux  Inputs=3
  Scope1 : Scope
      settings: ActiveDisplayYMinimum=-53.661197596804719  ActiveDisplayYMaximum=492.95077837124262  DataLoggingVariableName=ScopeData3
  Out1 : Outport
  tag scope: v5=global
  wires:
  Demux1/3 -> MATLAB Function/3(theta)
  Integrator/1 -> Mux1/1, Integrator3/1
  Demux1/4 -> MATLAB Function/4(psi)
  Demux1/1 -> MATLAB Function/1(force)
  Demux1/2 -> MATLAB Function/2(phi)
  In1/1 -> Demux1/1
  MATLAB Function/1(x_ddot) -> Integrator/1
  MATLAB Function/2(y_ddot) -> Integrator1/1
  Integrator1/1 -> Mux1/2, Integrator4/1
  MATLAB Function/3(z_ddot) -> Integrator2/1
  Integrator2/1 -> Mux1/3, Integrator5/1
  Mux/1 -> Out1/1
  Integrator4/1 -> Mux/2
  Integrator3/1 -> Mux/1
  Integrator5/1 -> Mux/3, Scope1/1
  Mux1/1 -> [v5]

== system Drone_Formation/Drone 5/Subsystem2/Uncontrolled_UAV1/Subsystem1 ==
  tau : Inport
  omega : Inport  Port=2
  Integrator{,1..2,5} (4 alike) : Integrator
  Integrator3 : Integrator  InitialCondition=pi/4
  Integrator4 : Integrator  InitialCondition=pi/6
  MATLAB Function : MATLAB Function  TreatAsAtomicUnit=on
  Mux : Mux  Inputs=3
  Out1 : Outport
  wires:
  MATLAB Function/1(phi_ddot) -> Integrator/1
  tau/1 -> MATLAB Function/1(tau)
  MATLAB Function/2(theta_ddot) -> Integrator1/1
  MATLAB Function/3(psi_ddot) -> Integrator2/1
  Integrator/1 -> Integrator3/1, MATLAB Function/2(phi_dot)
  Integrator1/1 -> Integrator4/1, MATLAB Function/3(theta_dot)
  Integrator2/1 -> Integrator5/1, MATLAB Function/4(psi_dot)
  Integrator4/1 -> Mux/2  "theta"
  Integrator3/1 -> Mux/1  "phi"
  Integrator5/1 -> Mux/3  "psi"
  Mux/1 -> Out1/1
  omega/1 -> MATLAB Function/5(omega)

== matlab function Drone_Formation/Drone 5/Subsystem/Kinematic ==
  data: p1_ddot output; u input
function p1_ddot = fcn(u)

    p1_ddot = u;

end

== matlab function Drone_Formation/Drone 5/MATLAB Function1 ==
  data: p_ref input; u output; v_ref input; a_ref input; p input; v input; psi_r output
function [u, psi_r] = fcn(p_ref, v_ref, a_ref, p, v)

    kp = 4;
    kv = 3;

    A_adj = ones(5,5) - eye(5);
    a_ij = 0.5;

    L = zeros(5,5);
    for i = 1:5
        for j = 1:5
            if i ~= j && A_adj(i,j) == 1
                L(i,i) = L(i,i) + a_ij;
                L(i,j) = -a_ij;
            end
        end
    end

    psi_r = atan2(p_ref(14,1), p_ref(13,1));

    ep = p_ref(13:15,1) - p(13:15,1);
    ev = v_ref(13:15,1) - v(13:15,1);

    a = kron(L,ones(3))*((p_ref - p) + (v_ref - v));

    u = kp*ep + kv*ev + a_ref(13:15,1) + a(13:15,1);

end

== matlab function Drone_Formation/Drone 1/Subsystem2/MATLAB Function ==
  data: u input; force output; psi input; phi_r output; theta_r output
function [force, phi_r, theta_r] = fcn(u, psi)
    m = 1.5; g = 9.8;

    ux = u(1)*m;
    uy = u(2)*m;
    uz = (u(3)-g)*m;

    force = m*sqrt(ux^2 + uy^2 + (uz+g)^2);
    phi_r = asin(m*(ux*sin(psi) - uy*cos(psi))/force);
    theta_r = atan((ux*cos(psi) + uy*sin(psi))/(uz+g));
end

== matlab function Drone_Formation/Drone 1/Subsystem2/Subsystem/Lower Control ==
  data: Q456 input size=3; tau_x output size=1; tau_y output size=1; tau_z output size=1; s456 input size=3
function [tau_x, tau_y, tau_z] = fcn(Q456, s456)

    Ix = 4.8e-3; Iy = 4.8e-3; Iz = 9.8e-3;
    a = 10;

    tau_x = Ix*(Q456(1) - 2*s456(1) - a*sign(s456(1)));
    tau_y = Iy*(Q456(2) - 2*s456(2) - a*sign(s456(2)));
    tau_z = Iz*(Q456(3) - 2*s456(3) - a*sign(s456(3)));

end

== matlab function Drone_Formation/Drone 1/Subsystem2/Uncontrolled_UAV1/MATLAB Function1 ==
  data: force output; w1 input; w2 input; w3 input; w4 input; tau_x output; tau_y output; tau_z output; omega output
function [force, tau_x, tau_y, tau_z, omega] = fcn(w1, w2, w3, w4)

    l = 0.2; b = 2.92e-6; d = 1.12e-7;

    force = b*(w1^2 + w2^2 + w3^2 + w4^2);
    tau_x = l*b*(w4^2 - w2^2);
    tau_y = l*b*(w3^2 - w1^2);
    tau_z = d*(w2^2 + w4^2 - w1^2 - w3^2);
    omega = w1 + w3 - w2 - w4;

end

== matlab function Drone_Formation/Drone 1/Subsystem2/Uncontrolled_UAV1/Subsystem/MATLAB Function ==
  data: force input; x_ddot output; phi input; theta input; psi input; y_ddot output; z_ddot output
function [x_ddot, y_ddot, z_ddot] = fcn(force, phi, theta, psi)

    m = 1.5; g = 9.8;

    x_ddot = force*(cos(phi)*sin(theta)*cos(psi) + sin(phi)*sin(psi))/m;
    y_ddot = force*(cos(phi)*sin(theta)*sin(psi) - sin(phi)*cos(psi))/m;
    z_ddot = force*(cos(phi)*cos(theta))/m - g;

end

== matlab function Drone_Formation/Drone 1/Subsystem2/Uncontrolled_UAV1/Subsystem1/MATLAB Function ==
  data: tau input; phi_ddot output; phi_dot input; theta_dot input; psi_dot input; theta_ddot output; psi_ddot output; omega input
function [phi_ddot, theta_ddot, psi_ddot] = fcn(tau, phi_dot, theta_dot, psi_dot, omega)

    Ix = 4.8e-3; Iy = 4.8e-3; Iz = 9.8e-3;
    Jr = 1.287e-4;

    phi_ddot = (theta_dot*psi_dot*(Iy - Iz) - Jr*theta_dot*omega) + 1/Ix*tau(1);
    theta_ddot = (phi_dot*psi_dot*(Iz - Ix) + Jr*phi_dot*omega) + 1/Iy*tau(2);
    psi_ddot = (theta_dot*phi_dot*(Ix - Iy))/Iz + 1/Iz*tau(3);

end

== matlab function Drone_Formation/Drone 1/Subsystem2/Subsystem/MATLAB Function ==
  data: angle_dot input; e_dot input size=3; e input size=3; Q456 output size=3; s456 output; omega input size=1; angle_r_ddot input size=3
function [Q456, s456] = fcn(angle_dot, e_dot, e, omega, angle_r_ddot)

    Ix = 4.8e-3; Iy = 4.8e-3; Iz = 9.8e-3;
    Jr = 1.287e-4;
    b = 10;

    Q456 = zeros(3,1);
    s456 = zeros(3,1);

    s456(1) = b*e(1) + e_dot(1);
    s456(2) = b*e(2) + e_dot(2);
    s456(3) = b*e(3) + e_dot(3);

    Q456(1) = -b*e_dot(1) + angle_r_ddot(1) - angle_dot(2)*angle_dot(3)*(Iy - Iz)/Ix - Jr*angle_dot(2)*omega/Ix;
    Q456(2) = -b*e_dot(2) + angle_r_ddot(2) - angle_dot(1)*angle_dot(3)*(Iz - Ix)/Iy + Jr*angle_dot(1)*omega/Iy;
    Q456(3) = -b*e_dot(3) + angle_r_ddot(3) - angle_dot(1)*angle_dot(2)*(Ix - Iy)/Iz;


end

== matlab function Drone_Formation/Drone 1/Subsystem2/MATLAB Function1 ==
  data: force input; w output; tau input; u output
function [w,u] = fcn(force, tau)

    l = 0.2; b = 2.92e-6; d = 1.12e-7;

    A = [b, b, b, b;
         0, -l*b, 0, l*b;
         -l*b, 0, l*b, 0;
         -d, d, -d, d];
    u = [force; tau(1); tau(2); tau(3)];
    w1 = A\u;
    w = sqrt(abs(w1));
    
end

== matlab function Drone_Formation/Drone 1/Subsystem2/MATLAB Function2 ==
  data: u input; y output
function y = fcn(u)
    
    y = u(1) + u(3) - u(2) - u(4);

end

== matlab function Drone_Formation/Drone 2/Subsystem2/MATLAB Function ==
  data: u input; force output; psi input; phi_r output; theta_r output
function [force, phi_r, theta_r] = fcn(u, psi)
    m = 1.5; g = 9.8;

    ux = u(1)*m;
    uy = u(2)*m;
    uz = (u(3)-g)*m;

    force = m*sqrt(ux^2 + uy^2 + (uz+g)^2);
    phi_r = asin(m*(ux*sin(psi) - uy*cos(psi))/force);
    theta_r = atan((ux*cos(psi) + uy*sin(psi))/(uz+g));
end

== matlab function Drone_Formation/Drone 2/Subsystem2/MATLAB Function1 ==
  data: force input; w output; tau input; u output
function [w,u] = fcn(force, tau)

    l = 0.2; b = 2.92e-6; d = 1.12e-7;

    A = [b, b, b, b;
         0, -l*b, 0, l*b;
         -l*b, 0, l*b, 0;
         -d, d, -d, d];
    u = [force; tau(1); tau(2); tau(3)];
    w1 = A\u;
    w = sqrt(abs(w1));
    
end

== matlab function Drone_Formation/Drone 2/Subsystem2/MATLAB Function2 ==
  data: u input; y output
function y = fcn(u)
    
    y = u(1) + u(3) - u(2) - u(4);

end

== matlab function Drone_Formation/Drone 2/Subsystem2/Subsystem/Lower Control ==
  data: Q456 input size=3; tau_x output size=1; tau_y output size=1; tau_z output size=1; s456 input size=3
function [tau_x, tau_y, tau_z] = fcn(Q456, s456)

    Ix = 4.8e-3; Iy = 4.8e-3; Iz = 9.8e-3;
    a = 10;

    tau_x = Ix*(Q456(1) - 2*s456(1) - a*sign(s456(1)));
    tau_y = Iy*(Q456(2) - 2*s456(2) - a*sign(s456(2)));
    tau_z = Iz*(Q456(3) - 2*s456(3) - a*sign(s456(3)));

end

== matlab function Drone_Formation/Drone 1/Subsystem1/Kinematic ==
  data: p1_ddot output; u input
function p1_ddot = fcn(u)

    p1_ddot = u;

end

== matlab function Drone_Formation/Drone 2/Subsystem2/Subsystem/MATLAB Function ==
  data: angle_dot input; e_dot input size=3; e input size=3; Q456 output size=3; s456 output; omega input size=1; angle_r_ddot input size=3
function [Q456, s456] = fcn(angle_dot, e_dot, e, omega, angle_r_ddot)

    Ix = 4.8e-3; Iy = 4.8e-3; Iz = 9.8e-3;
    Jr = 1.287e-4;
    b = 10;

    Q456 = zeros(3,1);
    s456 = zeros(3,1);

    s456(1) = b*e(1) + e_dot(1);
    s456(2) = b*e(2) + e_dot(2);
    s456(3) = b*e(3) + e_dot(3);

    Q456(1) = -b*e_dot(1) + angle_r_ddot(1) - angle_dot(2)*angle_dot(3)*(Iy - Iz)/Ix - Jr*angle_dot(2)*omega/Ix;
    Q456(2) = -b*e_dot(2) + angle_r_ddot(2) - angle_dot(1)*angle_dot(3)*(Iz - Ix)/Iy + Jr*angle_dot(1)*omega/Iy;
    Q456(3) = -b*e_dot(3) + angle_r_ddot(3) - angle_dot(1)*angle_dot(2)*(Ix - Iy)/Iz;


end

== matlab function Drone_Formation/Drone 2/Subsystem2/Uncontrolled_UAV1/MATLAB Function1 ==
  data: force output; w1 input; w2 input; w3 input; w4 input; tau_x output; tau_y output; tau_z output; omega output
function [force, tau_x, tau_y, tau_z, omega] = fcn(w1, w2, w3, w4)

    l = 0.2; b = 2.92e-6; d = 1.12e-7;

    force = b*(w1^2 + w2^2 + w3^2 + w4^2);
    tau_x = l*b*(w4^2 - w2^2);
    tau_y = l*b*(w3^2 - w1^2);
    tau_z = d*(w2^2 + w4^2 - w1^2 - w3^2);
    omega = w1 + w3 - w2 - w4;

end

== matlab function Drone_Formation/Drone 2/Subsystem2/Uncontrolled_UAV1/Subsystem/MATLAB Function ==
  data: force input; x_ddot output; phi input; theta input; psi input; y_ddot output; z_ddot output
function [x_ddot, y_ddot, z_ddot] = fcn(force, phi, theta, psi)

    m = 1.5; g = 9.8;

    x_ddot = force*(cos(phi)*sin(theta)*cos(psi) + sin(phi)*sin(psi))/m;
    y_ddot = force*(cos(phi)*sin(theta)*sin(psi) - sin(phi)*cos(psi))/m;
    z_ddot = force*(cos(phi)*cos(theta))/m - g;

end

== matlab function Drone_Formation/Drone 2/Subsystem2/Uncontrolled_UAV1/Subsystem1/MATLAB Function ==
  data: tau input; phi_ddot output; phi_dot input; theta_dot input; psi_dot input; theta_ddot output; psi_ddot output; omega input
function [phi_ddot, theta_ddot, psi_ddot] = fcn(tau, phi_dot, theta_dot, psi_dot, omega)

    Ix = 4.8e-3; Iy = 4.8e-3; Iz = 9.8e-3;
    Jr = 1.287e-4;

    phi_ddot = (theta_dot*psi_dot*(Iy - Iz) - Jr*theta_dot*omega) + 1/Ix*tau(1);
    theta_ddot = (phi_dot*psi_dot*(Iz - Ix) + Jr*phi_dot*omega) + 1/Iy*tau(2);
    psi_ddot = (theta_dot*phi_dot*(Ix - Iy))/Iz + 1/Iz*tau(3);

end

== matlab function Drone_Formation/Drone 3/Subsystem2/MATLAB Function ==
  data: u input; force output; psi input; phi_r output; theta_r output
function [force, phi_r, theta_r] = fcn(u, psi)
    m = 1.5; g = 9.8;

    ux = u(1)*m;
    uy = u(2)*m;
    uz = (u(3)-g)*m;

    force = m*sqrt(ux^2 + uy^2 + (uz+g)^2);
    phi_r = asin(m*(ux*sin(psi) - uy*cos(psi))/force);
    theta_r = atan((ux*cos(psi) + uy*sin(psi))/(uz+g));
end

== matlab function Drone_Formation/Drone 3/Subsystem2/MATLAB Function1 ==
  data: force input; w output; tau input; u output
function [w,u] = fcn(force, tau)

    l = 0.2; b = 2.92e-6; d = 1.12e-7;

    A = [b, b, b, b;
         0, -l*b, 0, l*b;
         -l*b, 0, l*b, 0;
         -d, d, -d, d];
    u = [force; tau(1); tau(2); tau(3)];
    w1 = A\u;
    w = sqrt(abs(w1));
    
end

== matlab function Drone_Formation/Virtual Trajectory/MATLAB Function ==
  data: t input; p_ref output
function p_ref = fcn(t)

    R = 30; omega = 2; vz = 0.5;

    offset = 5;
    offset_body = [0, 0, 0;
                    offset, 0, 0;
                    -offset, 0, 0;
                    0, offset, 0;
                    0, -offset, 0];

    x = R*cos(omega*t);
    y = R*sin(omega*t);
    z = vz*t;

    psi = atan2(y,x);

    R = [cos(psi), -sin(psi), 0;
        sin(psi), cos(psi), 0;
        0, 0, 1];

    p1 = [x; y; z];
    p2 = p1 + R*offset_body(2,:)';
    p3 = p1 + R*offset_body(3,:)';
    p4 = p1 + R*offset_body(4,:)';
    p5 = p1 + R*offset_body(5,:)';

    p_ref = [p1; p2; p3; p4; p5];

end

== matlab function Drone_Formation/Drone 3/Subsystem2/MATLAB Function2 ==
  data: u input; y output
function y = fcn(u)
    
    y = u(1) + u(3) - u(2) - u(4);

end

== matlab function Drone_Formation/Drone 3/Subsystem2/Subsystem/Lower Control ==
  data: Q456 input size=3; tau_x output size=1; tau_y output size=1; tau_z output size=1; s456 input size=3
function [tau_x, tau_y, tau_z] = fcn(Q456, s456)

    Ix = 4.8e-3; Iy = 4.8e-3; Iz = 9.8e-3;
    a = 10;

    tau_x = Ix*(Q456(1) - 2*s456(1) - a*sign(s456(1)));
    tau_y = Iy*(Q456(2) - 2*s456(2) - a*sign(s456(2)));
    tau_z = Iz*(Q456(3) - 2*s456(3) - a*sign(s456(3)));

end

== matlab function Drone_Formation/Drone 3/Subsystem2/Subsystem/MATLAB Function ==
  data: angle_dot input; e_dot input size=3; e input size=3; Q456 output size=3; s456 output; omega input size=1; angle_r_ddot input size=3
function [Q456, s456] = fcn(angle_dot, e_dot, e, omega, angle_r_ddot)

    Ix = 4.8e-3; Iy = 4.8e-3; Iz = 9.8e-3;
    Jr = 1.287e-4;
    b = 10;

    Q456 = zeros(3,1);
    s456 = zeros(3,1);

    s456(1) = b*e(1) + e_dot(1);
    s456(2) = b*e(2) + e_dot(2);
    s456(3) = b*e(3) + e_dot(3);

    Q456(1) = -b*e_dot(1) + angle_r_ddot(1) - angle_dot(2)*angle_dot(3)*(Iy - Iz)/Ix - Jr*angle_dot(2)*omega/Ix;
    Q456(2) = -b*e_dot(2) + angle_r_ddot(2) - angle_dot(1)*angle_dot(3)*(Iz - Ix)/Iy + Jr*angle_dot(1)*omega/Iy;
    Q456(3) = -b*e_dot(3) + angle_r_ddot(3) - angle_dot(1)*angle_dot(2)*(Ix - Iy)/Iz;


end

== matlab function Drone_Formation/Drone 3/Subsystem2/Uncontrolled_UAV1/MATLAB Function1 ==
  data: force output; w1 input; w2 input; w3 input; w4 input; tau_x output; tau_y output; tau_z output; omega output
function [force, tau_x, tau_y, tau_z, omega] = fcn(w1, w2, w3, w4)

    l = 0.2; b = 2.92e-6; d = 1.12e-7;

    force = b*(w1^2 + w2^2 + w3^2 + w4^2);
    tau_x = l*b*(w4^2 - w2^2);
    tau_y = l*b*(w3^2 - w1^2);
    tau_z = d*(w2^2 + w4^2 - w1^2 - w3^2);
    omega = w1 + w3 - w2 - w4;

end

== matlab function Drone_Formation/Drone 3/Subsystem2/Uncontrolled_UAV1/Subsystem/MATLAB Function ==
  data: force input; x_ddot output; phi input; theta input; psi input; y_ddot output; z_ddot output
function [x_ddot, y_ddot, z_ddot] = fcn(force, phi, theta, psi)

    m = 1.5; g = 9.8;

    x_ddot = force*(cos(phi)*sin(theta)*cos(psi) + sin(phi)*sin(psi))/m;
    y_ddot = force*(cos(phi)*sin(theta)*sin(psi) - sin(phi)*cos(psi))/m;
    z_ddot = force*(cos(phi)*cos(theta))/m - g;

end
